simulink model "Exercitiul_1"  (R2021b)
settings: Solver=VariableStepAuto  StartTime=0.0  StopTime=10.0  RelTol=1e-3
libraries: simulink x1
settings Model: Creator=Petrisor  LastModifiedBy=Petrisor

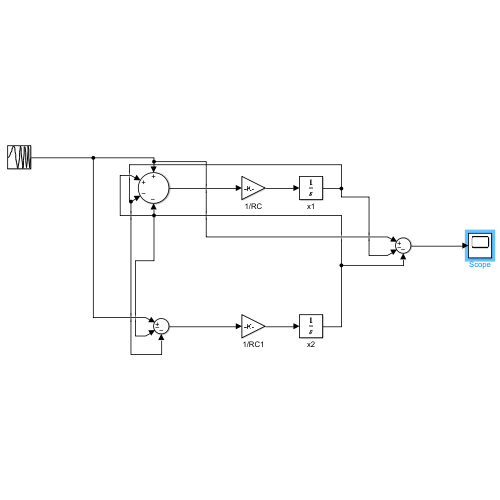
[thumbnail: Simulink's stored preview of the top-level diagram]
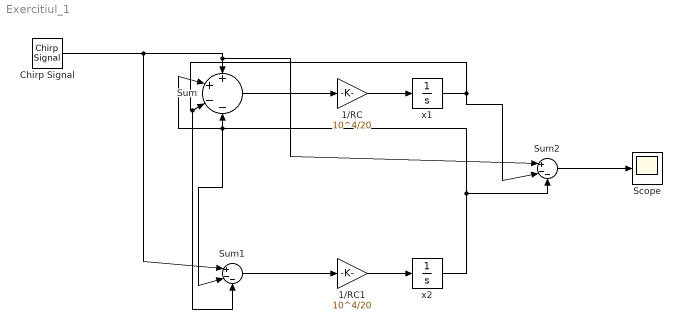
== system Exercitiul_1 ==
  1/RC : Gain  Gain=10^4/20
  1/RC1 : Gain  Gain=10^4/20
  Chirp Signal : simulink/Sources/Chirp Signal  f1=1  T=100  f2=100
  Scope : Scope
  Sum : Sum  Inputs=++--
  Sum1 : Sum  Inputs=|+--
  Sum2 : Sum  Inputs=|+--
  x1 : Integrator
  x2 : Integrator
  wires:
  Sum/1 -> 1/RC/1
  1/RC/1 -> x1/1
  Chirp Signal/1 -> Sum1/1, Sum2/1, Sum/1
  x2/1 -> Sum2/3, Sum/2, Sum/4, Sum1/2
  x1/1 -> Sum2/2, Sum1/3, Sum/3
  1/RC1/1 -> x2/1
  Sum1/1 -> 1/RC1/1
  Sum2/1 -> Scope/1
